simulink model "untitled1"  (R2023b)
settings: Solver=VariableStepAuto  StartTime=0.0  StopTime=50  RelTol=1e-3
values from neighbouring files (symbols this model uses):
  A = double(A_linear)    [main.m]    (also in rlqr.m = [0 1; -6 -5])
  B = double(B_linear)    [main.m]    (also in rlqr.m = [0;1])
undefined symbols (not defined in the file or in its folder): K1, K2
settings Model: Creator=ralex  LastModifiedBy=ralex

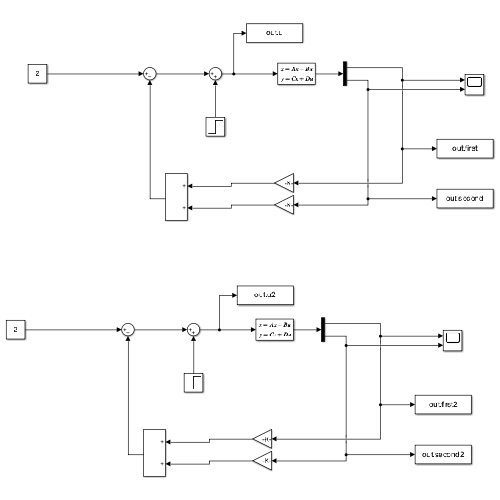
[thumbnail: Simulink's stored preview of the top-level diagram]
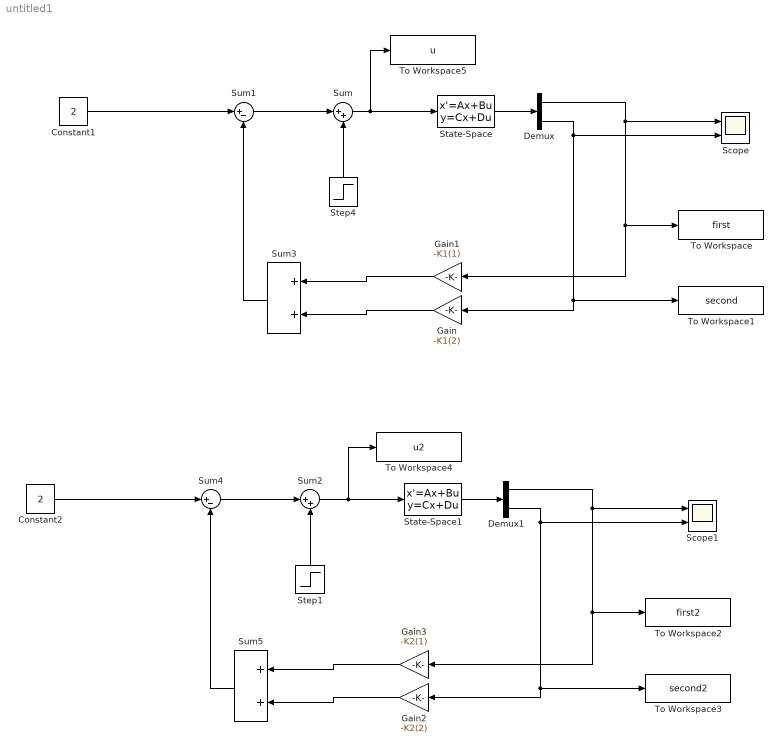
== system untitled1 ==
  Constant1 : Constant  Value=2
  Constant2 : Constant  Value=2
  Demux : Demux  Outputs=2
  Demux1 : Demux  Outputs=2
  Gain : Gain  Gain=-K1(2)
  Gain1 : Gain  Gain=-K1(1)
  Gain2 : Gain  Gain=-K2(2)
  Gain3 : Gain  Gain=-K2(1)
  Scope : Scope  NumInputPorts=2
  Scope1 : Scope  NumInputPorts=2
  State-Space : StateSpace  A=A  B=B  C=eye(2)  D=[0;0]  InitialCondition=[0 0]
  State-Space1 : StateSpace  A=A  B=B  C=eye(2)  D=[0;0]  InitialCondition=[0 0]
  Step1 : Step  Time=10  Before=2  After=3  SampleTime=0
  Step4 : Step  Time=10  Before=2  After=3  SampleTime=0
  Sum : Sum  Inputs=|++
  Sum1 : Sum  Inputs=|+-
  Sum2 : Sum  Inputs=|++
  Sum3 : Sum
  Sum4 : Sum  Inputs=|+-
  Sum5 : Sum
  To Workspace : ToWorkspace  VariableName=first  SaveFormat=Timeseries  SampleTime=-1
  To Workspace1 : ToWorkspace  VariableName=second  SaveFormat=Timeseries  SampleTime=-1
  To Workspace2 : ToWorkspace  VariableName=first2  SaveFormat=Timeseries  SampleTime=-1
  To Workspace3 : ToWorkspace  VariableName=second2  SaveFormat=Timeseries  SampleTime=-1
  To Workspace4 : ToWorkspace  VariableName=u2  SaveFormat=Timeseries  SampleTime=-1
  To Workspace5 : ToWorkspace  VariableName=u  SaveFormat=Timeseries  SampleTime=-1
  wires:
  Step4/1 -> Sum/2
  Sum3/1 -> Sum1/2
  Gain/1 -> Sum3/2
  Gain1/1 -> Sum3/1
  Demux/1 -> Gain1/1, To Workspace/1, Scope/1
  State-Space/1 -> Demux/1
  Demux/2 -> Gain/1, To Workspace1/1, Scope/2
  Sum1/1 -> Sum/1
  Constant1/1 -> Sum1/1
  Sum/1 -> To Workspace5/1, State-Space/1
  Constant2/1 -> Sum4/1
  Sum4/1 -> Sum2/1
  Sum2/1 -> To Workspace4/1, State-Space1/1
  Gain3/1 -> Sum5/1
  Demux1/1 -> Gain3/1, To Workspace2/1, Scope1/1
  State-Space1/1 -> Demux1/1
  Sum5/1 -> Sum4/2
  Step1/1 -> Sum2/2
  Gain2/1 -> Sum5/2
  Demux1/2 -> Gain2/1, To Workspace3/1, Scope1/2
